simulink library "rtwdemo_SimpleSchedModel"  (Simulink 7.6)
settings: Solver=ode45  SolverMode=SingleTasking  StartTime=0.0  StopTime=10.0  RelTol=1e-3
libraries: rtwdemo_SimpleSchedModel x1
settings Model: Creator=The MathWorks Inc.  ExtModeAutoUpdateStatusClock=off

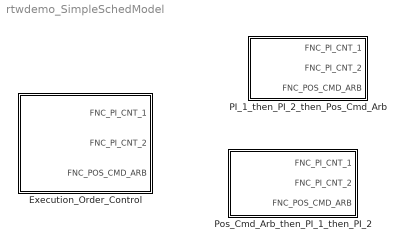
== system rtwdemo_SimpleSchedModel ==
  Execution_Order_Control : Subsystem  BlockChoice=PI_1_then_PI_2_then_Pos_Cmd_Arb
      settings: TemplateBlock=self  MemberBlocks=PI_1_then_PI_2_then_Pos_Cmd_Arb,Pos_Cmd_Arb_then_PI_1_then_PI_2
  PI_1_then_PI_2_then_Pos_Cmd_Arb : Subsystem  RTWFcnName=Scheduling_Model
      settings: RTWSystemCode=Function  RTWFcnNameOpts=User specified  RTWFileNameOpts=Use function name
  Pos_Cmd_Arb_then_PI_1_then_PI_2 : Subsystem  RTWFcnName=Scheduling_Model
      settings: MinAlgLoopOccurrences=on  RTWSystemCode=Function  RTWFcnNameOpts=User specified  RTWFileNameOpts=Use function name

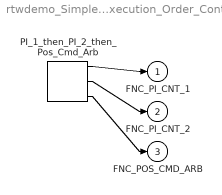
== system rtwdemo_SimpleSchedModel/Execution_Order_Control ==
  PI_1_then_PI_2_then_Pos_Cmd_Arb : rtwdemo_SimpleSchedModel/PI_1_then_PI_2_then_Pos_Cmd_Arb  SystemSampleTime=-1
  FNC_PI_CNT_1 : Outport
  FNC_PI_CNT_2 : Outport  Port=2
  FNC_POS_CMD_ARB : Outport  Port=3
  wires:
  PI_1_then_PI_2_then_Pos_Cmd_Arb/1 -> FNC_PI_CNT_1/1
  PI_1_then_PI_2_then_Pos_Cmd_Arb/2 -> FNC_PI_CNT_2/1
  PI_1_then_PI_2_then_Pos_Cmd_Arb/3 -> FNC_POS_CMD_ARB/1

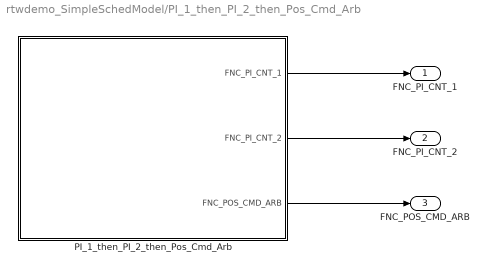
== system rtwdemo_SimpleSchedModel/PI_1_then_PI_2_then_Pos_Cmd_Arb ==
  PI_1_then_PI_2_then_Pos_Cmd_Arb : Stateflow chart  TreatAsAtomicUnit=on  SystemSampleTime=.001
  FNC_PI_CNT_1 : Outport
  FNC_PI_CNT_2 : Outport  Port=2
  FNC_POS_CMD_ARB : Outport  Port=3
  wires:
  PI_1_then_PI_2_then_Pos_Cmd_Arb/1(FNC_PI_CNT_1) -> FNC_PI_CNT_1/1
  PI_1_then_PI_2_then_Pos_Cmd_Arb/2(FNC_PI_CNT_2) -> FNC_PI_CNT_2/1
  PI_1_then_PI_2_then_Pos_Cmd_Arb/3(FNC_POS_CMD_ARB) -> FNC_POS_CMD_ARB/1

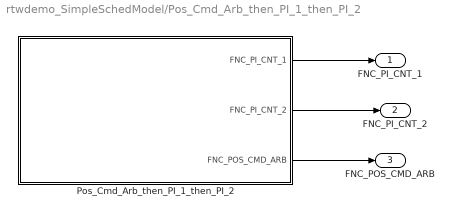
== system rtwdemo_SimpleSchedModel/Pos_Cmd_Arb_then_PI_1_then_PI_2 ==
  Pos_Cmd_Arb_then_PI_1_then_PI_2 : Stateflow chart  TreatAsAtomicUnit=on  SystemSampleTime=.001
  FNC_PI_CNT_1 : Outport
  FNC_PI_CNT_2 : Outport  Port=2
  FNC_POS_CMD_ARB : Outport  Port=3
  wires:
  Pos_Cmd_Arb_then_PI_1_then_PI_2/1(FNC_PI_CNT_1) -> FNC_PI_CNT_1/1
  Pos_Cmd_Arb_then_PI_1_then_PI_2/2(FNC_PI_CNT_2) -> FNC_PI_CNT_2/1
  Pos_Cmd_Arb_then_PI_1_then_PI_2/3(FNC_POS_CMD_ARB) -> FNC_POS_CMD_ARB/1

== stateflow chart PI_1_then_PI_2_then_Pos_Cmd_Arb/PI_1_then_PI_2_then_Pos_Cmd_Arb ==
  (default) -> (junction 3)
  (junction 3) -> (junction 4) : {
      | FNC_PI_CNT_1;
      | }
  (junction 4) -> (junction 5) : {
      | FNC_PI_CNT_2;
      | }
  (junction 5) -> (junction 6) : {
      | FNC_POS_CMD_ARB;
      | }
  (junction 6) -> (junction 7)
  events: FNC_PI_CNT_1 output FUNCTION_CALL_EVENT; FNC_PI_CNT_2 output FUNCTION_CALL_EVENT; FNC_POS_CMD_ARB output FUNCTION_CALL_EVENT

== stateflow chart Pos_Cmd_Arb_then_PI_1_then_PI_2/Pos_Cmd_Arb_then_PI_1_then_PI_2 ==
  (default) -> (junction 18)
  (junction 18) -> (junction 19) : {
      | FNC_POS_CMD_ARB;
      | }
  (junction 19) -> (junction 20) : {
      | FNC_PI_CNT_1;
      | }
  (junction 20) -> (junction 21) : {
      | FNC_PI_CNT_2;
      | }
  (junction 21) -> (junction 22)
  events: FNC_PI_CNT_1 output FUNCTION_CALL_EVENT; FNC_PI_CNT_2 output FUNCTION_CALL_EVENT; FNC_POS_CMD_ARB output FUNCTION_CALL_EVENT
